simulink model "model"  (R2023b)
settings: Solver=VariableStepAuto  StartTime=0.0  StopTime=600  RelTol=1e-3
values from neighbouring files (symbols this model uses):
  aT = 0    [data.m]
  gamma0 = 0    [data.m]
  gammaT = 0    [data.m]
  N = 3    [data.m]
  Rhit = 3    [data.m]
  Tc = 0.1    [data.m]
  V = 300    [data.m]
  Vc = 400    [data.m]
  VT = 290    [data.m]
  Xt0 = 4000    [data.m]
  Yt0 = 2000    [data.m]
libraries: simulink x1
settings Model: PacingRate=4  Creator=aadit  LastModifiedBy=aadit

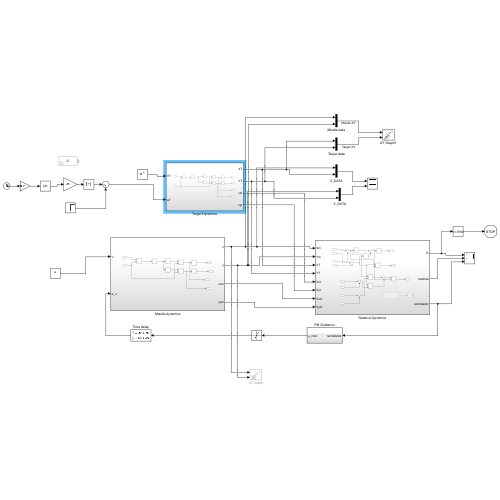
[thumbnail: Simulink's stored preview of the top-level diagram]
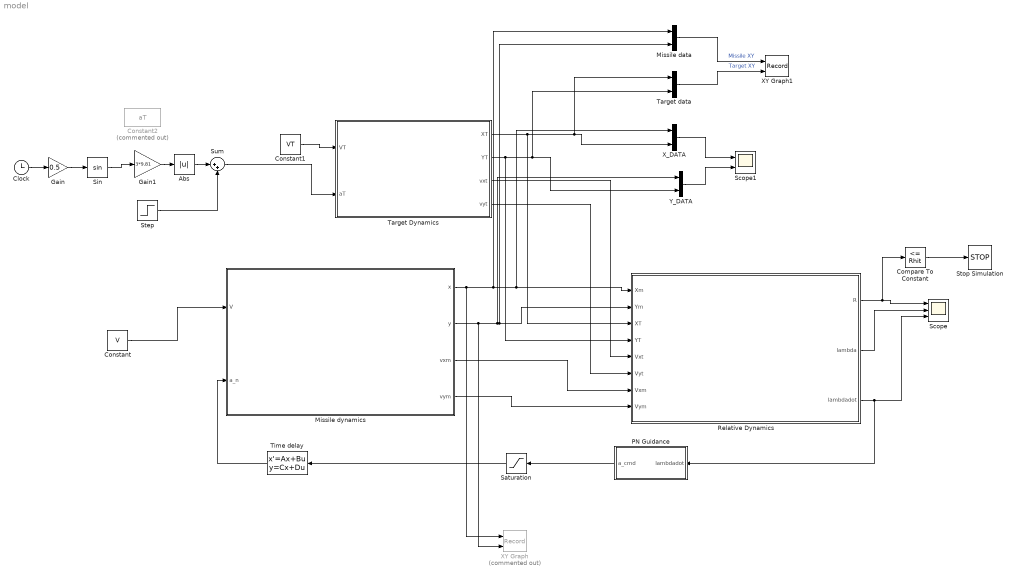
== system model ==
  Abs : Abs  SaturateOnIntegerOverflow=off
  Clock : Clock
  Compare To Constant : simulink/Logic and Bit Operations/Compare To Constant  relop=<=  const=Rhit  OutDataTypeStr=boolean
  Constant : Constant  Value=V
  Constant1 : Constant  Value=VT
  Constant2 : Constant  Commented=on  Value=aT
  Gain : Gain  Gain=0.5
  Gain1 : Gain  Gain=3*9.81
  Missile data : Mux  Inputs=2
  Missile dynamics : Subsystem
  PN Guidance : Subsystem
  Relative Dynamics : Subsystem
  Saturation : Saturate  UpperLimit=30*9.81  LowerLimit=-30*9.81
  Scope : Scope  NumInputPorts=3
  Scope1 : Scope  NumInputPorts=2
  Sin : Trigonometry
  Step : Step  Time=10  After=3*9.81  SampleTime=0
  Stop Simulation : Stop
  Sum : Sum  Inputs=|++
  Target Dynamics : Subsystem
  Target data : Mux  Inputs=2
  Time delay : StateSpace  A=-1/Tc  B=1/Tc  D=0  InitialCondition=0
  XY Graph : Record  Commented=on  FileSettingsInternal="{\"entries\":[{\"content\":{\"excelSettings\":{\"content\":{},\"type\":\"Streamout.ExcelSettings\"}},\"type\":\"Streamout.FileSettingStorage\",\"uuid\":\"\"}],\"packageUris\":[\"http:\\/\\/schema.mathworks.com\\/mf0\\/streamout_blocks\\/R2020a\"],\"version\":\"1.0\"}"  Layout=[1 1]  SignalsInternal="{\"entries\":[{\"content\":{\"signals\":[{\"content\":{\"blockPath\":[],\"dimensions\":[1],\"domain\":\"\",\"lineColor\":\"#fe330a\",\"port\":1,\"signalID\":1,\"signalName\":\"Missile dynamics:1\"},\"type\":\"RecordBlkView.Signal\",\"uuid\":\"\"},{\"content\":{\"blockPath\":[],\"dimensions\":[1],\"domain\":\"\",\"lineColor\":\"#22b573\",\"port\":2,\"signalID\":2,\"signalName\":\"Missile dynamics:2\"},\"type\":\"RecordBlkView.Signal\",\"uuid\":\"\"}]},\"type\":\"RecordBlkView.InputSignals\",\"uuid\":\"\"}],\"packageUris\":[\"http:\\/\\/schema.mathworks.com\\/mf0\\/streamout_blocks\\/R2020a\"],\"version\":\"1.0\"}"  CompatibilityTag=XY
  XY Graph1 : Record  VariableName=interception  FileSettingsInternal="{\"entries\":[{\"content\":{\"excelSettings\":{\"content\":{},\"type\":\"Streamout.ExcelSettings\"}},\"type\":\"Streamout.FileSettingStorage\",\"uuid\":\"\"}],\"packageUris\":[\"http:\\/\\/schema.mathworks.com\\/mf0\\/streamout_blocks\\/R2020a\"],\"version\":\"1.0\"}"  Layout=[1 1]  SignalsInternal="{\"entries\":[{\"content\":{\"signals\":[{\"content\":{\"blockPath\":[],\"dimensions\":[2],\"domain\":\"\",\"hasChildren\":true,\"lineColor\":\"#77ac30\",\"port\":1,\"sid\":[\"\"],\"signalID\":1,\"signalName\":\"Missile XY\"},\"type\":\"RecordBlkView.Signal\",\"uuid\":\"\"},{\"content\":{\"blockPath\":[],\"channel\":[1],\"dimensions\":[2],\"domain\":\"\",\"lineColor\":\"#4dbeee\",\"parentID\":1,\"port\":1,\"sid\":[\"\"],\"signalID\":2,\"signalName\":\"Missile XY\"},\"type\":\"RecordBlkView.Signal\",\"uuid\":\"\"},{\"content\":{\"blockPath\":[],\"dimensions\":[2],\"domain\":\"\",\"hasChildren\":true,\"lineColor\":\"#a2142f\",\"port\":2,\"sid\":[\"\"],\"signalID\":3,\"signalName\":\"Target XY\"},\"type\":\"RecordBlkView.Signal\",\"uuid\":\"\"},{\"content\":{\"blockPath\":[],\"channel\":[1],\"dimensions\":[2],\"domain\":\"\",\"lineColor\":\"#139fff\",\"parentID\":3,\"port\":2,\"sid\":[\"\"],\"signalID\":4,\"signalName\":\"Target XY\"},\"type\":\"RecordBlkView.Signal\",\"uuid\":\"\"},{\"content\":{\"blockPath\":[],\"channel\":[2],\"dimensions\":[2],\"domain\":\"\",\"lineColor\":\"#ff6929\",\"parentID\":1,\"port\":1,\"sid\":[\"\"],\"signalID\":5,\"signalName\":\"Missile XY\"},\"type\":\"RecordBlkView.Signal\",\"uuid\":\"\"},{\"content\":{\"blockPath\":[],\"channel\":[2],\"dimensions\":[2],\"domain\":\"\",\"lineColor\":\"#b746ff\",\"parentID\":3,\"port\":2,\"sid\":[\"\"],\"signalID\":6,\"signalName\":\"Target XY\"},\"type\":\"RecordBlkView.Signal\",\"uuid\":\"\"}]},\"type\":\"RecordBlkView.InputSignals\",\"uuid\":\"\"}],\"packageUris\":[\"http:\\/\\/schema.mathworks.com\\/mf0\\/streamout_blocks\\/R2020a\"],\"version\":\"1.0\"}"  CompatibilityTag=XY
  X_DATA : Mux  Inputs=2
  Y_DATA : Mux  Inputs=2
  wires:
  Missile dynamics/1(x) -> X_DATA/1, Relative Dynamics/1(Xm), Missile data/1, XY Graph/1
  Missile dynamics/2(y) -> Missile data/2, Relative Dynamics/2(Ym), Y_DATA/1, XY Graph/2
  Constant/1 -> Missile dynamics/1(V)
  Relative Dynamics/1(R) -> Compare To Constant/1, Scope/1
  Relative Dynamics/2(lambda) -> Scope/2
  Relative Dynamics/3(lambdadot) -> Scope/3, PN Guidance/1(lambdadot)
  PN Guidance/1(a_cmd) -> Saturation/1
  Compare To Constant/1 -> Stop Simulation/1
  Time delay/1 -> Missile dynamics/2(a_n)
  Saturation/1 -> Time delay/1
  Constant1/1 -> Target Dynamics/1(VT)
  Target Dynamics/1(XT) -> X_DATA/2, Target data/1, Relative Dynamics/3(XT)
  Target Dynamics/2(YT) -> Y_DATA/2, Target data/2, Relative Dynamics/4(YT)
  Y_DATA/1 -> Scope1/2
  X_DATA/1 -> Scope1/1
  Missile data/1 -> XY Graph1/1  "Missile XY"
  Target data/1 -> XY Graph1/2  "Target XY"
  Clock/1 -> Gain/1
  Gain/1 -> Sin/1
  Sin/1 -> Gain1/1
  Step/1 -> Sum/2
  Sum/1 -> Target Dynamics/2(aT)
  Missile dynamics/3(vxm) -> Relative Dynamics/7(Vxm)
  Missile dynamics/4(vym) -> Relative Dynamics/8(Vym)
  Target Dynamics/3(vxt) -> Relative Dynamics/5(Vxt)
  Target Dynamics/4(vyt) -> Relative Dynamics/6(Vyt)
  Gain1/1 -> Abs/1
  Abs/1 -> Sum/1

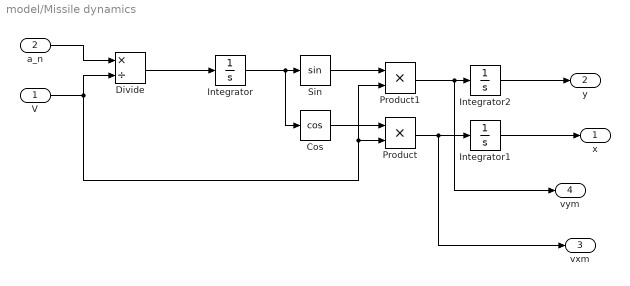
== system model/Missile dynamics ==
  V : Inport
  a_n : Inport  Port=2
  Cos : Trigonometry  Operator=cos
  Divide : Product  Inputs=*/
  Integrator : Integrator  InitialCondition=gamma0
  Integrator1 : Integrator
  Integrator2 : Integrator  InitialCondition=1000
  Product : Product
  Product1 : Product
  Sin : Trigonometry
  x : Outport
  y : Outport  Port=2
  vxm : Outport  Port=3
  vym : Outport  Port=4
  wires:
  V/1 -> Divide/2, Product/2, Product1/2
  Divide/1 -> Integrator/1
  Integrator/1 -> Cos/1, Sin/1
  Cos/1 -> Product/1
  Sin/1 -> Product1/1
  Integrator2/1 -> y/1
  Integrator1/1 -> x/1
  a_n/1 -> Divide/1
  Product/1 -> vxm/1, Integrator1/1
  Product1/1 -> vym/1, Integrator2/1

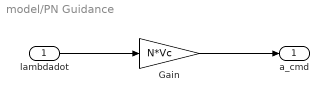
== system model/PN Guidance ==
  lambdadot : Inport
  Gain : Gain  Gain=N*Vc
  a_cmd : Outport
  wires:
  lambdadot/1 -> Gain/1
  Gain/1 -> a_cmd/1

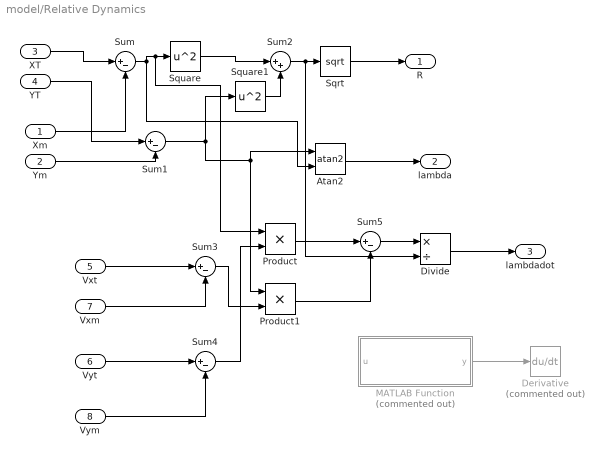
== system model/Relative Dynamics ==
  Xm : Inport
  Ym : Inport  Port=2
  XT : Inport  Port=3
  YT : Inport  Port=4
  Vxt : Inport  Port=5
  Vyt : Inport  Port=6
  Vxm : Inport  Port=7
  Vym : Inport  Port=8
  Atan2 : Trigonometry  Operator=atan2
  Derivative : Derivative  Commented=on
  Divide : Product  Inputs=*/
  MATLAB Function : MATLAB Function  Commented=on  TreatAsAtomicUnit=on
  Product : Product
  Product1 : Product
  Sqrt : Sqrt
  Square : Math  Operator=square
  Square1 : Math  Operator=square
  Sum{,1,3..5} (5 alike) : Sum  Inputs=|+-
  Sum2 : Sum  Inputs=|++
  R : Outport
  lambda : Outport  Port=2
  lambdadot : Outport  Port=3
  wires:
  XT/1 -> Sum/1
  Xm/1 -> Sum/2
  YT/1 -> Sum1/1
  Ym/1 -> Sum1/2
  Sum/1 -> Product/1, Square/1, Atan2/2
  Sum1/1 -> Square1/1, Product1/1, Atan2/1
  Sum2/1 -> Divide/2, Sqrt/1
  Sqrt/1 -> R/1
  Atan2/1 -> lambda/1
  Square/1 -> Sum2/1
  Square1/1 -> Sum2/2
  Vxt/1 -> Sum3/1
  Vxm/1 -> Sum3/2
  Vyt/1 -> Sum4/1
  Vym/1 -> Sum4/2
  Sum4/1 -> Product/2
  Sum3/1 -> Product1/2
  Product/1 -> Sum5/1
  Product1/1 -> Sum5/2
  Sum5/1 -> Divide/1
  Divide/1 -> lambdadot/1
  MATLAB Function/1(y) -> Derivative/1

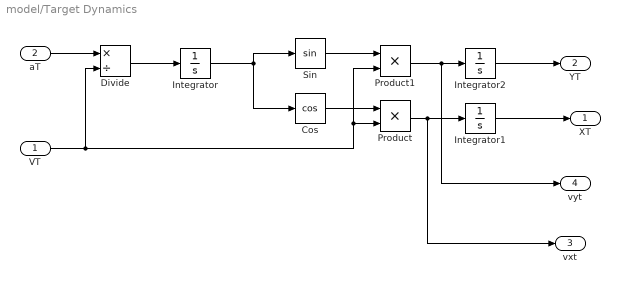
== system model/Target Dynamics ==
  VT : Inport
  aT : Inport  Port=2
  Cos : Trigonometry  Operator=cos
  Divide : Product  Inputs=*/
  Integrator : Integrator  InitialCondition=gammaT
  Integrator1 : Integrator  InitialCondition=Xt0
  Integrator2 : Integrator  InitialCondition=Yt0
  Product : Product
  Product1 : Product
  Sin : Trigonometry
  XT : Outport
  YT : Outport  Port=2
  vxt : Outport  Port=3
  vyt : Outport  Port=4
  wires:
  Integrator2/1 -> YT/1
  Integrator1/1 -> XT/1
  Cos/1 -> Product/1
  VT/1 -> Divide/2, Product/2, Product1/2
  Sin/1 -> Product1/1
  aT/1 -> Divide/1
  Divide/1 -> Integrator/1
  Integrator/1 -> Cos/1, Sin/1
  Product/1 -> vxt/1, Integrator1/1
  Product1/1 -> vyt/1, Integrator2/1

== matlab function model/Relative Dynamics/MATLAB Function ==
  data: u input; y output
function y = unwrap_lambda(u)
y = u;
    if (u < 0)
        y = u + 2*pi;
    end
end
